simulink model "SyC_Main"  (R2016b)
settings: configuration reference "CodeGenConfigSet" (kept outside this file)
undefined symbols (not defined in the file or in its folder): SyC_Main_DT
settings Model: Creator=zhoutinglin  LastModifiedBy=liutao
settings ConfigSetRef: SourceLocation=Base Workspace

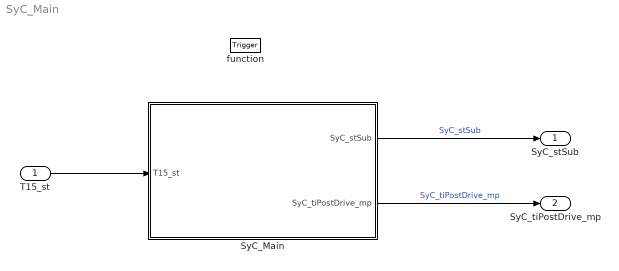
== system SyC_Main ==
  T15_st : Inport  Description=Terminal 15 status after debouncing  OutDataTypeStr=Enum: Switch_conv
  function : TriggerPort  TriggerType=function-call  VariantControl=Variant
  SyC_Main : Subsystem
  SyC_stSub : Outport  Description=Current system/ECU sub-state  OutDataTypeStr=Enum: SubSysExeState_conv
  SyC_tiPostDrive_mp : Outport  Tag=ms  Description=Afterrun time  Port=2  OutMin=0  OutMax=65535  OutDataTypeStr=Debounce_ms
  wires:
  SyC_Main/1(SyC_stSub) -> SyC_stSub/1  "SyC_stSub"
  T15_st/1 -> SyC_Main/1(T15_st)
  SyC_Main/2(SyC_tiPostDrive_mp) -> SyC_tiPostDrive_mp/1  "SyC_tiPostDrive_mp"

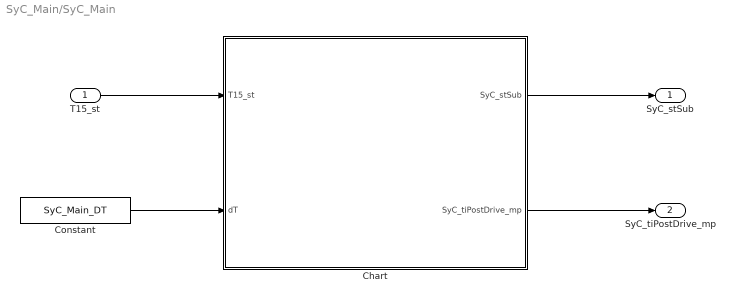
== system SyC_Main/SyC_Main ==
  T15_st : Inport
  Chart : Stateflow chart  TreatAsAtomicUnit=on
  Constant : Constant  Value=SyC_Main_DT
  SyC_stSub : Outport
  SyC_tiPostDrive_mp : Outport  Port=2
  wires:
  T15_st/1 -> Chart/1(T15_st)
  Chart/1(SyC_stSub) -> SyC_stSub/1
  Constant/1 -> Chart/2(dT)
  Chart/2(SyC_tiPostDrive_mp) -> SyC_tiPostDrive_mp/1

== stateflow chart SyC_Main/Chart ==
  state PreDrive
    entry:
    SyC_stSub=SubSysExeState_conv.SYC_PREDRIVE
  state Drive
    entry:
    SyC_stSub=SubSysExeState_conv.SYC_DRIVE
  state PostDrive
    entry:
    SyC_stSub=SubSysExeState_conv.SYC_POSTDRIVE;
    SyC_tiPostDrive_mp=dT;
    during:
    SyC_tiPostDrive_mp=SyC_tiPostDrive_mp+dT;
    exit:
    SyC_tiPostDrive_mp=0;
  (default) -> PreDrive
  PreDrive -> Drive : [T15_st==1]
  PostDrive -> PreDrive [order 2] : [(T15_st==0) && (SyC_tiPostDrive_mp>=SyC_tiPostDrive_C)]
  Drive -> PostDrive : [T15_st==0]
  PostDrive -> Drive [order 1] : [T15_st==1]
  data: T15_st input; SyC_stSub output; dT input; SyC_tiPostDrive_mp output; SyC_tiPostDrive_C parameter
